simulink model "sim_all"  (R2020a)
settings: Solver=VariableStepAuto  StartTime=0.0  StopTime=2000  RelTol=1e-3
values from neighbouring files (symbols this model uses):
  nav_DT = 0.1    [navigation.m]
  nav_giro = 2    [navigation.m]
  nav_h0 = 0    [navigation.m]
  nav_lat0 = cornerC(1)    [navigation.m]
  nav_lon0 = cornerC(2)    [navigation.m]
  nav_plane_AB = coefficient_plane(nav_A,nav_B)    [navigation.m]
  nav_plane_BC = coefficient_plane(nav_B,nav_C)    [navigation.m]
  nav_plane_CD = coefficient_plane(nav_C,nav_D)    [navigation.m]
  nav_plane_DA = coefficient_plane(nav_D,nav_A)    [navigation.m]
undefined symbols (not defined in the file or in its folder): a1, a2, alpha1, alpha2, cornerA, cornerB, cornerC, cornerD, ctrl_clockwise, ctrl_int_bound_or, ctrl_int_bound_pos, ctrl_k_or, ctrl_k_pos, ctrl_Ki_vel, ctrl_Kp_v_pos, ctrl_Kp_vel, ctrl_TAM, ctrl_Ts, ctrl_va_uncontrolled, ctrl_vel_uncontrolled, D, dead_zone_limit, depth, DiscIntNeverNeededParam, distanceFromWall, initInspectedSide, initPoint, mod_A, mod_Cd_F, mod_Cd_M, mod_eta_init, mod_g, mod_h0, mod_Ixx, mod_Iyy, mod_Izz, mod_Kp_dot, mod_lat0, mod_lon0, mod_m, mod_Mq_dot, mod_ni_init, mod_Nr_dot, mod_p1, mod_p2, mod_p3, mod_p4, mod_p5, mod_p6, mod_R, mod_Rm, mod_t1, mod_t2, mod_t3, mod_t4, mod_t5, mod_t6, mod_W, mod_Xu_dot, mod_Yv_dot ... (+44)
libraries: simulink x8, cstblocks x6, simulink_extras x1
(part 6 of 6)

== matlab function sim_all/Sensors/Environment1 ==
  data: plane_AB output; plane_BC output; plane_CD output; plane_DA output; plane_W output
function [plane_AB,plane_BC,plane_CD,plane_DA,plane_W] = fcn()
%% Inizializzazione
% Coordinate degli spigoli del bacino in lat e long fornite dal file
% missionC.m
A= zeros(1,3);
B= zeros(1,3);
C= zeros(1,3);
D= zeros(1,3);
cornerA = [43.781381; 11.282793]; % Lat/Lon [decimal degrees]      
cornerB = [43.780975; 11.283505]; % Lat/Lon [decimal degrees]       
cornerC = [43.780189; 11.282698]; % Lat/Lon [decimal degrees]       
cornerD = [43.780602; 11.281956]; % Lat/Lon [decimal degrees]

% Definizione terna NED con origine (lat0,long0,h0) coincidente al 
% cornerD
coder.extrinsic('evalin', 'wgs84Ellipsoid', 'geodetic2ned');
lat0 = cornerC(1);
lon0 = cornerC(2);
h0 = 0;

%% Conversione ECEF to NED
[A(1),A(2),A(3)] = geodetic2ned(cornerA(1),cornerA(2),0,lat0,lon0,h0,wgs84Ellipsoid);
[B(1),B(2),B(3)] = geodetic2ned(cornerB(1),cornerB(2),0,lat0,lon0,h0,wgs84Ellipsoid);
[C(1),C(2),C(3)] = geodetic2ned(cornerC(1),cornerC(2),0,lat0,lon0,h0,wgs84Ellipsoid);
[D(1),D(2),D(3)] = geodetic2ned(cornerD(1),cornerD(2),0,lat0,lon0,h0,wgs84Ellipsoid);

%% Calcolo delle distanze dalle pareti
% L'equazione del piano corrisponde a quella della retta perché il piano
% delle pareti è verticale, per cui si risolve un sistema lineare:
% l'equazione del piano deve soddisfare il passaggio da due punti.
% Il parametro a è libero, lo poniamo a=1, il parametro c relativo all'asse
% z sarà sempre pari a zero.

% questo è il sistema da risolvere
b = - (B(1)- A(1)) /( B(2) - A(2) );   %AB
d = - A(1) - A(2)*b;

e = - (C(1)-B(1))/(C(2)-B(2));         %BC
f = - B(1) - B(2)*e;

g = - (D(1) - C(1)) / (D(2) - C(2));   %CD
h = - C(1) - C(2)*g;

i = - (A(1) - D(1))/(A(2) - D(2));     %DA
l = -D(1) - D(2)*i;

% syms b d;
% [b d] = solve(A(1)+b*A(2)+d,B(1)+b*B(2)+d,b,d);
a_AB = 1;
b_AB = double(b);
c_AB = 0;
d_AB = double(d);
% 
% syms b d ;
% [b d] = solve(B(1)+b*B(2)+d,C(1)+b*C(2)+d,b,d);
a_BC = 1;
b_BC = double(e);
c_BC = 0;
d_BC = double(f);

a_CD = 1;
b_CD = double(g);
c_CD = 0;
d_CD = double(h);

a_DA = 1;
b_DA = double(i);
c_DA = 0;
d_DA = double(l);


% calcolo dei coefficienti del piano direttamente con la formula esplicita
plane_AB = [a_AB b_AB c_AB d_AB];
plane_BC = [a_BC b_BC c_BC d_BC];
plane_CD = [a_CD b_CD c_CD d_CD];
plane_DA = [a_DA b_DA c_DA d_DA];
plane_W =[0 0 1 0];

== matlab function sim_all/Sensors/GEOD to NED1 ==
  data: z output; lat input; lon input; h input
function z  = fcn(lat,lon,h)
z=[0;0;0];
coder.extrinsic('evalin','wgs84Ellipsoid','geodetic2ned');
[N,E,D] = geodetic2ned(lat,lon,h,43.780189,11.282698,0,wgs84Ellipsoid);
z=[N;E;D];

== matlab function sim_all/Sensors/NED to GEOD1 ==
  data: z output; N input; E input
function z  = fcn(N,E)
z=zeros(2,1);
coder.extrinsic('evalin','wgs84Ellipsoid','ned2geodetic');
%profondità considerata come solo antenna GPS fuori dall'acqua
[LAT,LON,~]=ned2geodetic(N,E,-0.385,43.780189,11.282698,0,wgs84Ellipsoid);
z=[LAT;LON];

== matlab function sim_all/Model/from Rad to Deg ==
  data: eta2 input; eta2_deg output
function eta2_deg = fcn(eta2)

phi = eta2(1);
theta = eta2(2);
psi = eta2(3);

% Si effettua una conversione da radianti a gradi dell'angolo di roll:
k_phi = fix(phi/(2*pi));
orientation_phi = phi - (2*pi*k_phi);
phi_deg = (180*orientation_phi)/pi;

% Si effettua una conversione da radianti a gradi dell'angolo di pitch:
k_theta = fix(theta/(2*pi));
orientation_theta = theta - (2*pi*k_theta);
theta_deg = (180*orientation_theta)/pi;

% Si effettua una conversione da radianti a gradi dell'angolo di yaw:
k_psi = fix(psi/(2*pi));
orientation_psi = psi - (2*pi*k_psi);
psi_deg = (180*orientation_psi)/pi;

% Se si vuole mostrare anche il numero di rotazioni che compie il robot in
% roll, pitch o yaw mandare in uscita anche k_phi, k_theta e k_psi.

eta2_deg = [phi_deg; theta_deg; psi_deg];

== matlab function sim_all/Controller_mk4_v3/signal_to_NED/Signal_d->NED/ToNed ==
  data: vel input; ddp input; dps input; orp input; vel_n output size=[3 1]; wall_vect input; wall_vect2 input; state input; ctrl_clockwise parameter; ddp_n output size=[3 1]; dps_n output size=[3 1]; orp_n output size=[3 1]
%% A partire dai riferimenti scalari calcola i relativi vettori in terna NED
function [vel_n,ddp_n,dps_n,orp_n] = ToNed(vel, ddp, dps, orp, wall_vect, wall_vect2, state, ctrl_clockwise)
    w=wall_vect/norm(wall_vect);        % versore relativo alla pareta che stiamo pattugliando
    n = Cz(-pi/2)*wall_vect;            % vettore ortogonale entrante dalla parete in pattugliamento
    n=n/norm(n);                        % versore ortogonale alla parete in pattugliamento
    n2 = Cz(-pi/2)*wall_vect2;          % vettore ortogonale entrante dalla parete successiva
    n2=n2/norm(n2);                     % versore ortogonale alla parete successiva
    if ctrl_clockwise == true           % la velocità dipende dalla direzione di pattugliamento
        vel_n=w*vel;                    % stessa direzione della parete
    else
        vel_n=-w*vel;
    end
    ddp_n = n*ddp;                          % vettore distanza dalla parete in pattugliamento in ned
    dps_n = n2*dps;                         % vettore distanza dalla parete successiva in ned
    v_orp = -n;                             % deve essere uscente dal bacino
    v_orp = Cz(-orp)*v_orp;                 % ruoto dell' angolo di riferimento
    orp_n=[0;0;atan2(v_orp(2),v_orp(1))];   % angolo rispetto all'asse x della terna ned
    if(state == 203)                        % orp_n deve essere relativo alla parete successiva
        v_orp = -n2;
        v_orp = Cz(-orp)*v_orp;
        orp_n=[0;0;atan2(v_orp(2),v_orp(1))];
    end
end

== matlab function sim_all/Controller_mk4_v3/signal_to_NED/Signal_d->NED/wall_fcn ==
  data: wall_vect output; WALL input; cornerA parameter; cornerB parameter; cornerC parameter; cornerD parameter; wall_vect2 output; ctrl_clockwise parameter
%% Restituisce i vettori Parete in pattugliamento e Parete successiva
function [wall_vect, wall_vect2] = wall_fcn(WALL,cornerA, cornerB, cornerC, cornerD, ctrl_clockwise) %inspectionDirection
    AB = zeros(3,1);
    BC = zeros(3,1);
    CD = zeros(3,1);
    DA = zeros(3,1);
    a = zeros(3,1);
    b = zeros(3,1);
    c = zeros(3,1);
    d = zeros(3,1);
    coder.extrinsic('evalin', 'wgs84Ellipsoid', 'geodetic2ned');
    [aNorth,aEast,aDown] = geodetic2ned(cornerA(1),cornerA(2),0,cornerC(1),cornerC(2),0,wgs84Ellipsoid);
    [bNorth,bEast,bDown] = geodetic2ned(cornerB(1),cornerB(2),0,cornerC(1),cornerC(2),0,wgs84Ellipsoid);
    [cNorth,cEast,cDown] = geodetic2ned(cornerC(1),cornerC(2),0,cornerC(1),cornerC(2),0,wgs84Ellipsoid);
    [dNorth,dEast,dDown] = geodetic2ned(cornerD(1),cornerD(2),0,cornerC(1),cornerC(2),0,wgs84Ellipsoid);
    a=[aNorth;aEast;aDown];
    b=[bNorth;bEast;bDown];
    c=[cNorth;cEast;cDown];
    d=[dNorth;dEast;dDown];
    AB = b-a;
    BC = c-b;
    CD = d-c;
    DA = a-d;
    if WALL == 1
        wall_vect = AB;
        if ctrl_clockwise == true
            wall_vect2 = BC;
        else
            wall_vect2 = DA;
        end
    elseif WALL == 2
        wall_vect = BC;
        if ctrl_clockwise == true
            wall_vect2 = CD;
        else
            wall_vect2 = AB;
        end
    elseif  WALL == 3
        wall_vect = CD;
        if ctrl_clockwise == true
            wall_vect2 = DA;
        else
            wall_vect2 = BC;
        end
    else   
        wall_vect = DA;
        if ctrl_clockwise == true
            wall_vect2 = AB;
        else
            wall_vect2 = CD;
        end
    end
end

== matlab function sim_all/Controller_mk4_v3/C_or/eta_dot2ni ==
  data: eta_dot input; or input; va output
%% Da NED a BODY
function va = fcn(eta_dot, or)

phi= or(1);
theta= or(2); 
psi= or(3);

J2inv = [[1;0;0], Cx(phi)*[0;1;0], Cx(phi)*Cy(theta)*[0;0;1]];
va = J2inv * eta_dot;
end

== matlab function sim_all/Mission_supervisor_v3/Mission_Supervisor/MATLAB Function ==
  data: parete_iniziale input; verso input; parete output; contatore input; initInspectedSide parameter; current_state input; giro output
function [parete, giro] = aggiorna_parete(parete_iniziale, verso, contatore, initInspectedSide,current_state)
   
 %% Corpo funzione 
    
    % A seconda del senso di pattugliamento si ha l'aggiornamento del valore
    % di parete attuale. 
    
    if(strcmp(verso,'clockwise') == 1)
        giro = 0;
        parete = mod((parete_iniziale + contatore),4);
        if(parete == 0)
            parete = 4;
        end
    else % 'counterclockwise'
        giro = 1;
        parete = parete_iniziale - contatore;
        if(parete <= 0)
            parete = parete+4;
        end
    end

    % Per stati precedenti al 201, si forza questa variabile a
    % mantenere il valore pari al valore iniziale. 
    if(current_state < 201)
        parete = initInspectedSide;
    end
    
end

== matlab function sim_all/Controller_mk4_v3/signal_to_NED/Signal_s->NED/ToNed ==
  data: ddp input; dps input; wall_vect input; ddp_n output size=[3 1]; dps_n output size=[3 1]; wall_vect2 input
%% A partire dalle stime scalari calcola i relativi vettori in terna NED
function [ddp_n,dps_n] = ToNed_s(ddp, dps,wall_vect, wall_vect2)
    n = Cz(-pi/2)*wall_vect;            % vettore ortogonale entrante dalla parete in pattugliamento
    n=n/norm(n);                        % versore ortogonale alla parete in pattugliamento
    n2 = Cz(-pi/2)*wall_vect2;          % vettore ortogonale entrante dalla parete successiva
    n2=n2/norm(n2);                     % versore ortogonale alla parete successiva
    ddp_n = n*ddp;                      % vettore distanza dalla parete in pattugliamento in ned
    dps_n = n2*dps;                     % vettore distanza dalla parete successiva in ned
end

== matlab function sim_all/Controller_mk4_v3/signal_to_NED/Signal_s->NED/wall_fcn1 ==
  data: wall_vect output; WALL input; cornerA parameter; cornerB parameter; cornerC parameter; cornerD parameter; wall_vect2 output; ctrl_clockwise parameter
%% Restituisce i vettori Parete in pattugliamento e Parete successiva
function [wall_vect, wall_vect2] = wall_fcn(WALL,cornerA, cornerB, cornerC, cornerD, ctrl_clockwise) %inspectionDirection
    AB = zeros(3,1);
    BC = zeros(3,1);
    CD = zeros(3,1);
    DA = zeros(3,1);
    a = zeros(3,1);
    b = zeros(3,1);
    c = zeros(3,1);
    d = zeros(3,1);
    coder.extrinsic('evalin', 'wgs84Ellipsoid', 'geodetic2ned');
    [aNorth,aEast,aDown] = geodetic2ned(cornerA(1),cornerA(2),0,cornerC(1),cornerC(2),0,wgs84Ellipsoid);
    [bNorth,bEast,bDown] = geodetic2ned(cornerB(1),cornerB(2),0,cornerC(1),cornerC(2),0,wgs84Ellipsoid);
    [cNorth,cEast,cDown] = geodetic2ned(cornerC(1),cornerC(2),0,cornerC(1),cornerC(2),0,wgs84Ellipsoid);
    [dNorth,dEast,dDown] = geodetic2ned(cornerD(1),cornerD(2),0,cornerC(1),cornerC(2),0,wgs84Ellipsoid);
    a=[aNorth;aEast;aDown];
    b=[bNorth;bEast;bDown];
    c=[cNorth;cEast;cDown];
    d=[dNorth;dEast;dDown];
    AB = b-a;
    BC = c-b;
    CD = d-c;
    DA = a-d;
    if WALL == 1
        wall_vect = AB;
        if ctrl_clockwise == true
            wall_vect2 = BC;
        else
            wall_vect2 = DA;
        end
    elseif WALL == 2
        wall_vect = BC;
        if ctrl_clockwise == true
            wall_vect2 = CD;
        else
            wall_vect2 = AB;
        end
    elseif  WALL == 3
        wall_vect = CD;
        if ctrl_clockwise == true
            wall_vect2 = DA;
        else
            wall_vect2 = BC;
        end
    else   
        wall_vect = DA;
        if ctrl_clockwise == true
            wall_vect2 = AB;
        else
            wall_vect2 = CD;
        end
    end
end

== matlab function sim_all/Controller_mk4_v3/signal_to_NED/prof_trigger ==
  settings: updateMethod=DISCRETE  sampleTime=ctrl_Ts
  data: state input; trigg_prof output
%% Trigger per la gestione dei segnali
% 1 se siamo in superficie
% 0 se siamo in profondità
function trigg_prof = fcn(state)
tmp = 0;
switch state
    case 100            % fermo in superficie
        tmp = 1;
    case 101            % orientazione verso parete di inizio in superficie
        tmp = 1;
    case 102            % posizionamento in superficie
        tmp = 1;   
    case 103            % immersione
        tmp = 1;
    case 104            % orientazione in profondità
        tmp = 0;
    case 201            % pattugliamento
        tmp = 0;
    case 202            % frenata
        tmp = 0;
    case 203            % manovra di cambio parete
        tmp = 0;
    case 204            % competamento del pattugliamento della parete iniziale
        tmp = 0;
    case 205            % frenata a metà parete
        tmp = 0;
    case 301            % risalita
        tmp = 0;
    case 302            % orientazione in superficie
        tmp = 1;
    case 303            % rientro, ritorno al punto iniziale in superficie
        tmp = 1;
    case 304            % fine missione, tutto spento
        tmp = 1;
end
trigg_prof = tmp;
end

== matlab function sim_all/Navigation/Calcolo distaza pareti/Calcolo distanza dalle pareti ==
  data: pos_es input; dpp output; dps output; parete_attuale input; nav_plane_AB parameter; nav_plane_BC parameter; nav_plane_CD parameter; nav_plane_DA parameter; nav_giro parameter
% Applicando la formula della distanza di un punto da un piano si ottiene la
% distanza della posizione dell'AUV dalla parete d'interesse. 

function [dpp,dps] = dpp_dps_calculator(pos_es, parete_attuale, nav_plane_AB, nav_plane_BC, nav_plane_CD, nav_plane_DA, nav_giro)
    
%selezione della parete di pattugliamento e successiva
    switch parete_attuale
        
        case 1
           coef = nav_plane_AB;            %parete attuale AB
           if nav_giro == 1
               coef_succ = nav_plane_BC;   %parete succ BC
           else
               coef_succ = nav_plane_DA;   %parete succ DA
           end
           
        case 2
           coef = nav_plane_BC;            %parete attuale BC
           if nav_giro == 1
               coef_succ = nav_plane_CD;   %parete succ CD
           else
               coef_succ = nav_plane_AB;   %parete succ AB
           end
           
        case 3
           coef = nav_plane_CD;            %parete attuale CD
           if nav_giro == 1
               coef_succ = nav_plane_DA;   %parete succ DA
           else
               coef_succ = nav_plane_BC;   %parete succ BC
           end
        case 4
           coef = nav_plane_DA;            %parete attuale DA
           if nav_giro == 1
               coef_succ = nav_plane_AB;   %parete succ AB
           else
               coef_succ = nav_plane_CD;   %parete succ CD
           end
        otherwise
            coef = [0 0 0 0];
            coef_succ = [0 0 0 0];
    end

    dpp = abs(coef(1)*pos_es(1)+coef(2)*pos_es(2)-coef(3)*pos_es(3)+coef(4))/norm([coef(1) coef(2) coef(3)]);
    dps = abs(coef_succ(1)*pos_es(1)+coef_succ(2)*pos_es(2)-coef_succ(3)*pos_es(3)+coef_succ(4))/norm([coef_succ(1) coef_succ(2) coef_succ(3)]);
   
end

== matlab function sim_all/Navigation/Calcolo distaza pareti/Calcolo orientazione dalla parete ==
  data: pos_es input; orient_parete output; parete_attuale input; orient input; nav_plane_AB parameter; nav_plane_BC parameter; nav_plane_CD parameter; nav_plane_DA parameter
function orient_parete  = orient_parete_calculator(pos_es, parete_attuale, orient, nav_plane_AB, nav_plane_BC, nav_plane_CD, nav_plane_DA)
    
    %consideriamo angoli di pitch e roll nulli, cioè si calcola
    %l'orientazione rispetto alla parete solo considerando rotazioni di yaw
    %(piano xy)

    Yaw   = orient(3);
    R_z = [cos(Yaw)     sin(Yaw)       0     ;
           -sin(Yaw)    cos(Yaw)       0     ;
              0            0           1    ];
    v_pos= R_z'*[1 0 0]';  %versore della retta lungo l'asse x (in body) in NED,
                       %cioè la direzione di riferimento di prua del veicolo     
    
    %selezione della parete di pattugliamento
switch parete_attuale                      
    case 1
        %% Piano di pattugliamento AB
        versore_plane_NED = [nav_plane_AB(1) nav_plane_AB(2) 0]';    %versore normale al piano
        versore_plane_NED = versore_plane_NED/norm(versore_plane_NED);

        %calcolo distanza e intersezione lungo la normale al piano
        t_ = -(pos_es(1)+nav_plane_AB(2)*pos_es(2)+nav_plane_AB(4))/(nav_plane_AB(2)*versore_plane_NED(2)+versore_plane_NED(1));
        inter_perp=zeros(3,1);
        inter_perp(1) = pos_es(1) + versore_plane_NED(1)*t_;
        inter_perp(2) = pos_es(2) + versore_plane_NED(2)*t_;
        inter_perp(3) = pos_es(3) + versore_plane_NED(3)*t_;
        
        %calcolo distanza e intersezione lungo la direzione di prua
        t_ = -(pos_es(1)+nav_plane_AB(2)*pos_es(2)+nav_plane_AB(4))/(nav_plane_AB(2)*v_pos(2)+v_pos(1));
        inter_prua=zeros(3,1);
        inter_prua(1) = pos_es(1) + v_pos(1)*t_;
        inter_prua(2) = pos_es(2) + v_pos(2)*t_;
        inter_prua(3) = pos_es(3) + v_pos(3)*t_;
        
        coef = nav_plane_AB;
        coef(4)=[];
        orient_parete = rad2deg(asin(abs(coef*v_pos)/(norm(coef)*norm(v_pos))));
        %se orient_parete è positiva, allora ci si trova tra - 90 e + 90 rispetto alla normale della parete 
        if t_ > 0              
            if inter_prua(1) > inter_perp(1) && inter_prua(2) < inter_perp(2)
                orient_parete = orient_parete - 90;
            else
                orient_parete = -(orient_parete - 90);
            end
        else
            if inter_prua(1) > inter_perp(1) && inter_prua(2) < inter_perp(2)
                orient_parete = (orient_parete + 90);
            else
                orient_parete = -(orient_parete + 90);
            end
        end    
    case 2
        %% Piano di pattugliamento BC
      	versore_plane_NED = [nav_plane_BC(1) nav_plane_BC(2) 0]';    %versore normale al piano
        versore_plane_NED = versore_plane_NED/norm(versore_plane_NED);

        %calcolo distanza e intersezione lungo la normale al piano
        t_ = -(pos_es(1)+nav_plane_BC(2)*pos_es(2)+nav_plane_BC(4))/(nav_plane_BC(2)*versore_plane_NED(2)+versore_plane_NED(1));
        inter_perp=zeros(3,1);
        inter_perp(1) = pos_es(1) + versore_plane_NED(1)*t_;
        inter_perp(2) = pos_es(2) + versore_plane_NED(2)*t_;
        inter_perp(3) = pos_es(3) + versore_plane_NED(3)*t_;

        %calcolo distanza e intersezione lungo la direzione di prua
        t_ = -(pos_es(1)+nav_plane_BC(2)*pos_es(2)+nav_plane_BC(4))/(nav_plane_BC(2)*v_pos(2)+v_pos(1));
        inter_prua=zeros(3,1);
        inter_prua(1) = pos_es(1) + v_pos(1)*t_;
        inter_prua(2) = pos_es(2) + v_pos(2)*t_;
        inter_prua(3) = pos_es(3) + v_pos(3)*t_;
        
        coef = nav_plane_BC;
        coef(4)=[];
        v_pos=-v_pos;
        orient_parete = rad2deg(asin(abs(coef*v_pos)/(norm(coef)*norm(v_pos))));
        %se orient_parete è positiva, allora ci si trova tra - 90 e + 90 rispetto alla normale della parete 
        if t_ > 0              
            if inter_prua(1) > inter_perp(1) && inter_prua(2) > inter_perp(2)
                orient_parete = orient_parete - 90;
            else
                orient_parete = -(orient_parete - 90);
            end
        else
            if inter_prua(1) > inter_perp(1) && inter_prua(2) > inter_perp(2)
                orient_parete = orient_parete + 90;
            else
                orient_parete = -(orient_parete + 90);
            end
        end
        
    case 3
        %% Piano di pattugliamento CD
      	versore_plane_NED = [nav_plane_CD(1) nav_plane_CD(2) 0]';    %versore normale al piano
        versore_plane_NED = versore_plane_NED/norm(versore_plane_NED);

        %calcolo distanza e intersezione lungo la normale al piano
        t_ = -(pos_es(1)+nav_plane_CD(2)*pos_es(2)+nav_plane_CD(4))/(nav_plane_CD(2)*versore_plane_NED(2)+versore_plane_NED(1));
        inter_perp=zeros(3,1);
        inter_perp(1) = pos_es(1) + versore_plane_NED(1)*t_;
        inter_perp(2) = pos_es(2) + versore_plane_NED(2)*t_;
        inter_perp(3) = pos_es(3) + versore_plane_NED(3)*t_;

        %calcolo distanza e intersezione lungo la direzione di prua
        t_ = -(pos_es(1)+nav_plane_CD(2)*pos_es(2)+nav_plane_CD(4))/(nav_plane_CD(2)*v_pos(2)+v_pos(1));
        inter_prua=zeros(3,1);
        inter_prua(1) = pos_es(1) + v_pos(1)*t_;
        inter_prua(2) = pos_es(2) + v_pos(2)*t_;
        inter_prua(3) = pos_es(3) + v_pos(3)*t_;
        
        coef = nav_plane_CD;
        coef(4)=[];
        v_pos=-v_pos;
        orient_parete = rad2deg(asin(abs(coef*v_pos)/(norm(coef)*norm(v_pos))));
        %se orient_parete è positiva, allora ci si trova tra - 90 e + 90 rispetto alla normale della parete 
        if t_ > 0              
            if inter_prua(1) > inter_perp(1) && inter_prua(2) < inter_perp(2)
                orient_parete = -orient_parete + 90;
            else
                orient_parete = orient_parete - 90;
            end
        else
             if inter_prua(1) > inter_perp(1) && inter_prua(2) < inter_perp(2)
                orient_parete = -orient_parete - 90;
            else
                orient_parete = orient_parete + 90;
            end
        end
        
    case 4
        %% Piano di pattugliamento DA
      	versore_plane_NED = [nav_plane_DA(1) nav_plane_DA(2) 0]';    %versore normale al piano
        versore_plane_NED = versore_plane_NED/norm(versore_plane_NED);

        %calcolo distanza e intersezione lungo la normale al piano
        t_ = -(pos_es(1)+nav_plane_DA(2)*pos_es(2)+nav_plane_DA(4))/(nav_plane_DA(2)*versore_plane_NED(2)+versore_plane_NED(1));
        inter_perp=zeros(3,1);
        inter_perp(1) = pos_es(1) + versore_plane_NED(1)*t_;
        inter_perp(2) = pos_es(2) + versore_plane_NED(2)*t_;
        inter_perp(3) = pos_es(3) + versore_plane_NED(3)*t_;

        %calcolo distanza e intersezione lungo la direzione di prua
        t_ = -(pos_es(1)+nav_plane_DA(2)*pos_es(2)+nav_plane_DA(4))/(nav_plane_DA(2)*v_pos(2)+v_pos(1));
        inter_prua=zeros(3,1);
        inter_prua(1) = pos_es(1) + v_pos(1)*t_;
        inter_prua(2) = pos_es(2) + v_pos(2)*t_;
        inter_prua(3) = pos_es(3) + v_pos(3)*t_;
        
        coef = nav_plane_DA;
        coef(4)=[];
        orient_parete = rad2deg(asin(abs(coef*v_pos)/(norm(coef)*norm(v_pos))));
        %se orient_parete è positiva, allora ci si trova tra - 90 e + 90 rispetto alla normale della parete 
        if t_ > 0              
            if inter_prua(1) < inter_perp(1) && inter_prua(2) < inter_perp(2)
                orient_parete = orient_parete - 90;
            else
                orient_parete = -orient_parete + 90;
            end
        else
            if inter_prua(1) < inter_perp(1) && inter_prua(2) < inter_perp(2)
                orient_parete = orient_parete + 90;
            else
                orient_parete = -orient_parete - 90;
            end
        end
        
    otherwise
        %%
       coef=[0 0 0 0];
       orient_parete = NaN;
end
    
    
end

== matlab function sim_all/Navigation/ECEF2NED ==
  data: GPS_ECEF input; GPS_NED output; nav_lat0 parameter; nav_lon0 parameter; nav_h0 parameter
%Componente di ingresso in terna ECEF
%Lat  [gradi]
%Long  [gradi]
%flag data_valid

function GPS_NED = GPS_conv_valid(GPS_ECEF, nav_lat0, nav_lon0, nav_h0)
    
    coder.extrinsic('evalin', 'wgs84Ellipsoid', 'geodetic2ned');

    if GPS_ECEF(3)==1
        GPS_NED = zeros(3,1);
        [GPS_NED(1),GPS_NED(2),GPS_NED(3)]= geodetic2ned(GPS_ECEF(1),GPS_ECEF(2),0,nav_lat0,nav_lon0,nav_h0,wgs84Ellipsoid);
        GPS_NED(3) = GPS_ECEF(3);
    else                            %qui non si effettua la conversione se il dato non è valido
        GPS_NED = GPS_ECEF; 
    end
end

== matlab function sim_all/Navigation/Extended Kalman Filter/AHRS__check/MATLAB Function4 ==
  data: flag_AHRS output; AHRS_new input; AHRS_now output; AHRS_old input
%gestione di misura errata di AHRS
function [flag_AHRS, AHRS_now] = fcn(AHRS_new, AHRS_old)

    if isnan(AHRS_new(1,1)) || isnan(AHRS_new(2,1)) || isnan(AHRS_new(3,1))
        AHRS_now = AHRS_old;
        flag_AHRS = 1;
        disp('Misura AHRS non valida')
    else
        AHRS_now = AHRS_new;
        flag_AHRS = 0;
    end  
end
